simulink model "MPC_Design"  (R2017a)
settings: Solver=VariableStepAuto  StartTime=0.0  StopTime=.3  MaxStep=1e-4  RelTol=1e-3
values from neighbouring files (symbols this model uses):
  G = [Gpp(1:p, 1:Nu) Gqp(1:p, 1:Nu) ; Gpq(1:p, 1:Nu) Gqq(1:p, 1:Nu)]    [DMC_initClalc.m]
  GF = [free(Yz(:, 1, 1), p, Nu) free(Yz(:, 1, 2), p, Nu);        free(Yz(:, 2, 1), p, Nu) free(Yz(:, 2, 2), p, Nu)]    [DMC_initClalc.m]
settings Model: Creator=erich  LastModifiedBy=erich

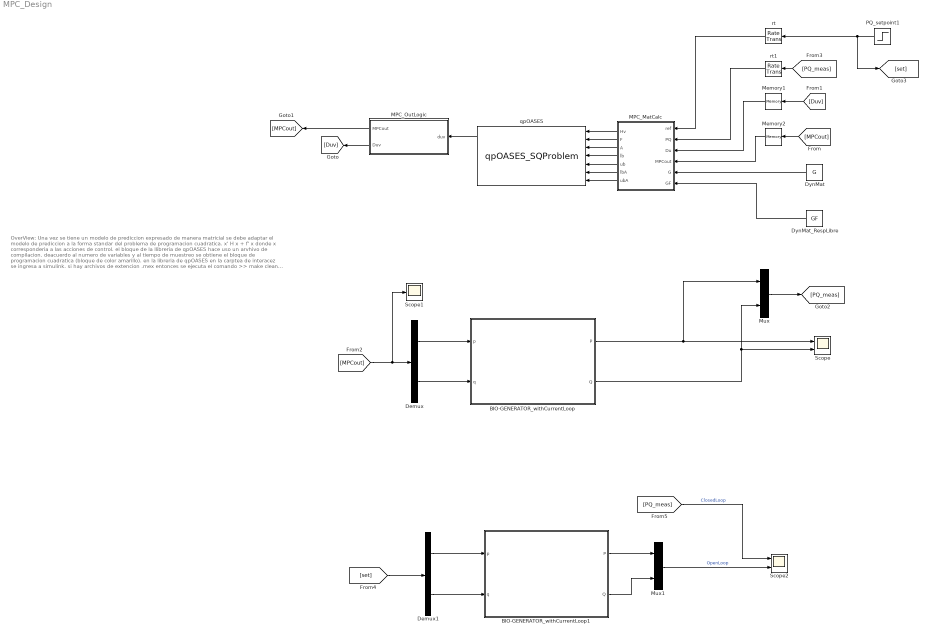
== system MPC_Design ==
  note: OverView:
      | Una vez se tiene un modelo de prediccion expresado de manera
      | matricial se debe adaptar el modelo de prediccion a la forma standar
      | del problema de programacion cuadratica.
      |
      | x' H x + f' x
      |
      | donde x corresponderia a las acciones de control.
      |
      | el bloque de la llibreria de qpOASES hace uso un arvhivo de compilacion.
      | deacuerdo al numero de variables y al tiempo de muestreo se obtiene el
      | bloque de programacion cuadratica (bloque de color amarillo).
      |
      | en la libreria de qpOASES en la carptea de interacez se ingresa a simulink.
      | si hay archivos de extencion .mex entonces se ejecuta el comando
      | >> make clean
      | para borrarlos.
      | se abre el archivo .cpp correspondiente a uno de los 3 bloques que se
      | desea usar de lla libreria (ver documentacion en la pagina oficial para
      | ver la diferencias entre cada uno de los bloques). una vez abierto el .cpp
      | se debe ubircar los #define donde se establece el timepo de muestreo y
      | el numero de variables a solucionar.
      | luego se ejecuta el comando:
      | >> make
      | luego se identifica .mex correspondiente al tipo de bloque que se desea
      | utilizar. este archivo debe estar en la misma carpeta del modelo de simulink
      | que va a hacer uso del bloque de qpOASES ya que el bloque de simulink
      | ejecuta sus funciones haciendo llamados al .mex
  BIO-GENERATOR_withCurrentLoop : Subsystem
  BIO-GENERATOR_withCurrentLoop1 : Subsystem
  Demux : Demux  Outputs=2
  Demux1 : Demux  Outputs=2
  DynMat : Constant  Value=G
  DynMat_RespLibre : Constant  Value=GF
  MPC_MatCalc : MATLAB Function  TreatAsAtomicUnit=on  SystemSampleTime=1e-3
      settings: MinAlgLoopOccurrences=on
  MPC_OutLogic : MATLAB Function  TreatAsAtomicUnit=on
      settings: MinAlgLoopOccurrences=on
  Memory1 : Memory
  Memory2 : Memory
  Mux : Mux  Inputs=2
  Mux1 : Mux  Inputs=2
  PQ_setpoint1 : Step  Time=[.1 .2]  Before=[0 0]  After=[500 2500]  SampleTime=0
  Scope : Scope  NumInputPorts=2
  Scope1 : Scope
  Scope2 : Scope  NumInputPorts=2
  qpOASES : S-Function  FunctionName=qpOASES_SQProblem  SFunctionDeploymentMode=off  EnableBusSupport=off
  rt : RateTransition  X0=[0 0]  OutPortSampleTime=1e-3
  rt1 : RateTransition  X0=[0 0]  OutPortSampleTime=1e-3
  wires:
  BIO-GENERATOR_withCurrentLoop/2(Q) -> Mux/2, Scope/2
  BIO-GENERATOR_withCurrentLoop/1(P) -> Scope/1, Mux/1
  Mux/1 -> [PQ_meas]
  MPC_MatCalc/1(Hv) -> qpOASES/1
  MPC_MatCalc/2(F) -> qpOASES/2
  MPC_MatCalc/3(A) -> qpOASES/3
  MPC_MatCalc/4(lb) -> qpOASES/4
  MPC_MatCalc/5(ub) -> qpOASES/5
  MPC_MatCalc/6(lbA) -> qpOASES/6
  MPC_MatCalc/7(ubA) -> qpOASES/7
  qpOASES/1 -> MPC_OutLogic/1(duv)
  MPC_OutLogic/2(Duv) -> [Duv]
  MPC_OutLogic/1(MPCout) -> [MPCout]
  [Duv] -> Memory1/1
  [MPCout] -> Memory2/1
  PQ_setpoint1/1 -> [set], rt/1
  rt/1 -> MPC_MatCalc/1(ref)
  Demux/1 -> BIO-GENERATOR_withCurrentLoop/1(p)
  Demux/2 -> BIO-GENERATOR_withCurrentLoop/2(" q")
  [MPCout] -> Scope1/1, Demux/1
  [PQ_meas] -> rt1/1
  rt1/1 -> MPC_MatCalc/2(PQ)
  DynMat/1 -> MPC_MatCalc/5(G)
  DynMat_RespLibre/1 -> MPC_MatCalc/6(GF)
  Memory1/1 -> MPC_MatCalc/3(Du)
  Memory2/1 -> MPC_MatCalc/4(MPCout)
  Demux1/1 -> BIO-GENERATOR_withCurrentLoop1/1(p)
  Demux1/2 -> BIO-GENERATOR_withCurrentLoop1/2(" q")
  [set] -> Demux1/1
  BIO-GENERATOR_withCurrentLoop1/1(P) -> Mux1/1
  BIO-GENERATOR_withCurrentLoop1/2(Q) -> Mux1/2
  Mux1/1 -> Scope2/2  "OpenLoop"
  [PQ_meas] -> Scope2/1  "ClosedLoop"

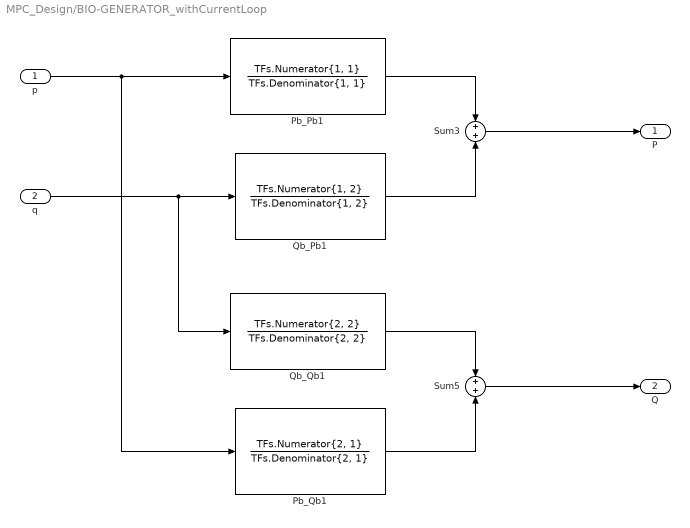
== system MPC_Design/BIO-GENERATOR_withCurrentLoop ==
  p : Inport
  " q" : Inport  Port=2
  Pb_Pb1 : TransferFcn  Numerator=TFs.Numerator{1, 1}  Denominator=TFs.Denominator{1, 1}
  Pb_Qb1 : TransferFcn  Numerator=TFs.Numerator{2, 1}  Denominator=TFs.Denominator{2, 1}
  Qb_Pb1 : TransferFcn  Numerator=TFs.Numerator{1, 2}  Denominator=TFs.Denominator{1, 2}
  Qb_Qb1 : TransferFcn  Numerator=TFs.Numerator{2, 2}  Denominator=TFs.Denominator{2, 2}
  Sum3 : Sum  Inputs=+|+
  Sum5 : Sum  Inputs=+|+
  P : Outport
  Q : Outport  Port=2
  wires:
  Qb_Pb1/1 -> Sum3/2
  Pb_Pb1/1 -> Sum3/1
  p/1 -> Pb_Pb1/1, Pb_Qb1/1
  Sum5/1 -> Q/1
  Pb_Qb1/1 -> Sum5/2
  Sum3/1 -> P/1
  Qb_Qb1/1 -> Sum5/1
  " q"/1 -> Qb_Pb1/1, Qb_Qb1/1

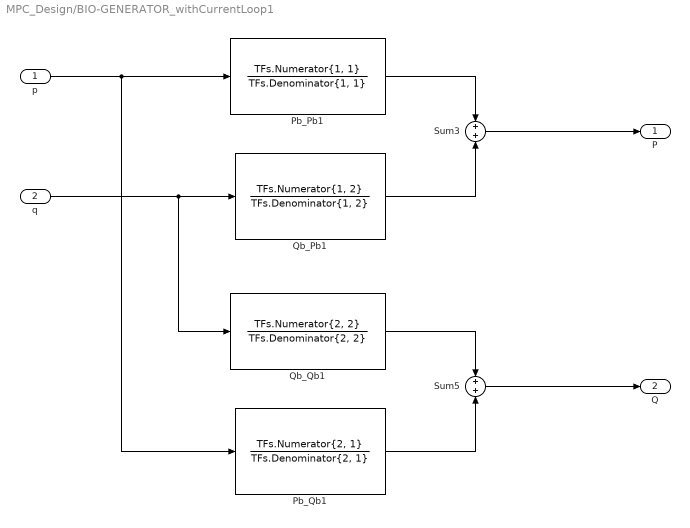
== system MPC_Design/BIO-GENERATOR_withCurrentLoop1 ==
  p : Inport
  " q" : Inport  Port=2
  Pb_Pb1 : TransferFcn  Numerator=TFs.Numerator{1, 1}  Denominator=TFs.Denominator{1, 1}
  Pb_Qb1 : TransferFcn  Numerator=TFs.Numerator{2, 1}  Denominator=TFs.Denominator{2, 1}
  Qb_Pb1 : TransferFcn  Numerator=TFs.Numerator{1, 2}  Denominator=TFs.Denominator{1, 2}
  Qb_Qb1 : TransferFcn  Numerator=TFs.Numerator{2, 2}  Denominator=TFs.Denominator{2, 2}
  Sum3 : Sum  Inputs=+|+
  Sum5 : Sum  Inputs=+|+
  P : Outport
  Q : Outport  Port=2
  wires:
  " q"/1 -> Qb_Qb1/1, Qb_Pb1/1
  Qb_Qb1/1 -> Sum5/1
  Sum3/1 -> P/1
  Pb_Qb1/1 -> Sum5/2
  Sum5/1 -> Q/1
  p/1 -> Pb_Qb1/1, Pb_Pb1/1
  Pb_Pb1/1 -> Sum3/1
  Qb_Pb1/1 -> Sum3/2

== matlab function MPC_Design/MPC_MatCalc ==
  data: ref input; PQ input; Hv output; F output; A output; lb output; ub output; lbA output; ubA output; Du input; MPCout input; G input; GF input
function [Hv, F, A, lb, ub, lbA, ubA] = MPC(ref, PQ, Du, MPCout, G, GF)

%%parametros del MPC


p = 100; % horizonte de prediccion
Nu = 100; % horizonte de control


%% Calculo de la salida de control.

H = G'*G+eye(2*Nu)*.1; % parte cuadratica del qp

ym = [ ones(p, 1)*PQ(1); ones(p, 1)*PQ(2) ]; % vector de la medida de tempearatura actual.

w = [ ones(p, 1)*ref(1); ones(p, 1)*ref(2) ]; % vector señal setpoint.

L = GF*Du+ym; % respuesta libre.

F = 2*(L-w)'*G; % parte lineal del problema qp.

A = zeros(1, 4*Nu*Nu);

lbA = zeros(1, 2*Nu);

ubA = zeros(1, 2*Nu);

Hv = M2V(H);

% % % % %
% CALCULO DE LAS RESTRICCIONES PARA EL Du
% % % % % 

% valores maximos y minimos para la salida del controlador
Pmax = 700;
Qmax = 4000;
Pmin = -700;
Qmin = -4000;

DPmax = 500;
DQmax = 1000;
DPmin = -500;
DQmin = -1000;


lb = [ones(1, Nu)*-1000 ones(1, Nu)*-2000];
ub = [ones(1, Nu)*1000 ones(1, Nu)*2000];

if ( MPCout(1) >= 0 )
    
    ub(1:Nu) = zeros(1, Nu);
else % si pa potencia activ de saldia es menor a 0
    
end
if ( MPCout(2) >= Qmax)
    lb = [zeros(1, Nu) zeros(1, Nu)];
end
lb = [ones(1, Nu)*-1000 ones(1, Nu)*-2000];
ub = [ones(1, Nu)*1000 ones(1, Nu)*2000];

== matlab function MPC_Design/MPC_OutLogic ==
  data: MPCout output; duv input; Duv output
function [MPCout, Duv] = MPC_out_Logic(duv)

%%parametros del MPC
Nu = 100; % horizonte de control.


%% variables del MPC
persistent Du; % deltas de u 
persistent out; % salida actual del conrolador MPC.

if isempty(Du) % inicializacion de los deltas de uu
    Du = zeros(2*Nu, 1);
end

if isempty(out) % inicializaion de la salida del controlador MPC
    out = [0; 0];
end


du = [duv(1), duv(Nu+1)];


Du = [du(1); Du(1:Nu-1); du(2); Du(Nu+1:end-1)];% actualizar historial deltas de u.

out = [ out(1)+du(1); out(2)+du(2) ]; %calcular salida del controlador.

MPCout = out;
Duv = Du;
